simulink model "plant_control_2"  (R2023a)
settings: Solver=FixedStepAuto  StartTime=0.0  StopTime=10.0  FixedStep=0.01  RelTol=1e-3
values from neighbouring files (symbols this model uses):
  attitude_ref = [15, 10, 0]    [control_law_design.m]
  g = 9.81    [control_law_design.m]
  Kp_p = 0.4858    [control_law_design.m]
  Kp_pitch = 14    [control_law_design.m]
  Kp_q = 0.4858    [control_law_design.m]
  Kp_r = 0.881    [control_law_design.m]
  Kp_roll = 14    [control_law_design.m]
  Kp_yaw = 12    [control_law_design.m]
  m = 0.468    [control_law_design.m]
libraries: simulink_extras x2, shared6dof x1
settings Model: Creator=timme  LastModifiedBy=timme
settings OptimizationCC: BlockReduction=off  DefaultParameterBehavior=Inlined  BufferReuse=off

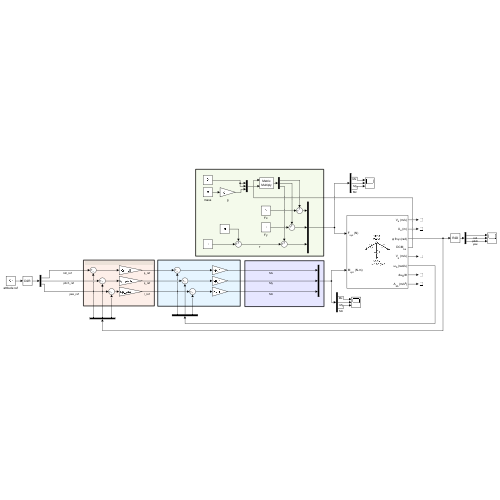
[thumbnail: Simulink's stored preview of the top-level diagram]
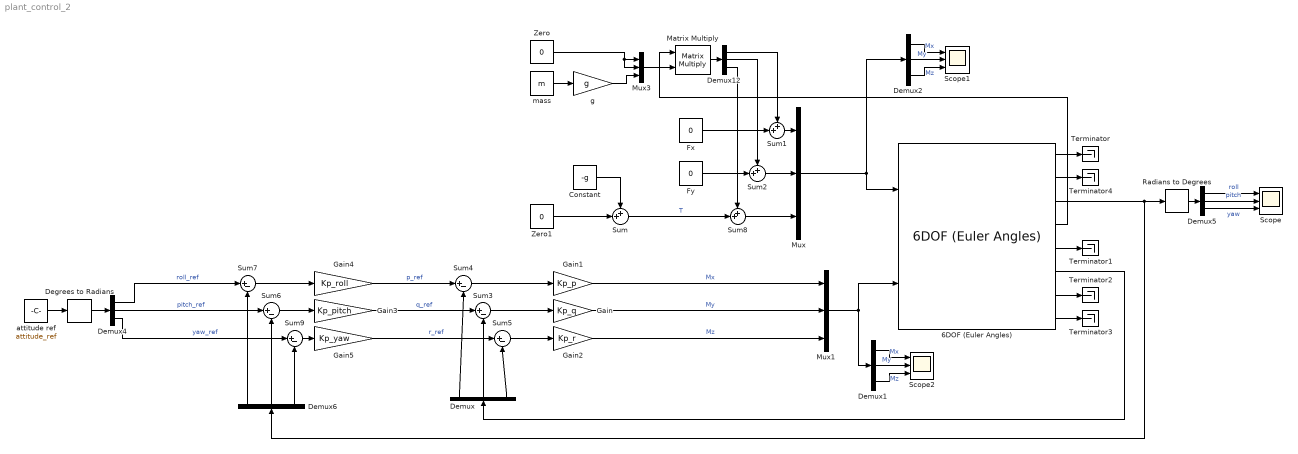
== system plant_control_2 ==
  6DOF (Euler Angles) : shared6dof/6DOF (Euler Angles)  units=Metric (MKS)  mtype=Fixed  rep=Euler Angles  xme_0=[0 0 0]  Vm_0=[0 0 0]  eul_0=[0 0 0]  pm_0=[0 0 0]  mass_0=m  mass_e=0.5  mass_f=2.0  inertia=I  inertia_e=eye(3)  inertia_f=2*eye(3)  k_quat=1.0  vre_flag=on  abi_flag=off  aMode=0  xme_statename=''  Vm_statename=''  eul_statename=''  quat_statename=''  pm_statename=''  mass_statename=''
  Constant : Constant  Value=-g
  Degrees to Radians : simulink_extras/Transformations/Degrees to Radians
  Demux{,1..2,4..6,12} (7 alike) : Demux  Outputs=3
  Fx : Constant  Value=0
  Fy : Constant  Value=0
  Gain : Gain  Gain=Kp_q
  Gain1 : Gain  Gain=Kp_p
  Gain2 : Gain  Gain=Kp_r
  Gain3 : Gain  Gain=Kp_pitch
  Gain4 : Gain  Gain=Kp_roll
  Gain5 : Gain  Gain=Kp_yaw
  Matrix Multiply : Product  Inputs=**  Multiplication=Matrix(*)
  Mux : Mux  Inputs=3
  Mux1 : Mux  Inputs=3
  Mux3 : Mux  Inputs=3
  Radians to Degrees : simulink_extras/Transformations/Radians to Degrees
  Scope : Scope  NumInputPorts=3
  Scope1 : Scope  NumInputPorts=3
  Scope2 : Scope  NumInputPorts=3
  Sum{,1..2,8} (4 alike) : Sum  Inputs=++|
  Sum{3..7,9} (6 alike) : Sum  Inputs=|+-
  Terminator{,1..4} (5 alike) : Terminator
  Zero : Constant  Value=0  OutDataTypeStr=Inherit: Inherit via back propagation
  Zero1 : Constant  Value=0  OutDataTypeStr=Inherit: Inherit via back propagation
  attitude ref : Constant  Value=attitude_ref
  g : Gain  Gain=g
  mass : Constant  Value=m
  wires:
  Mux1/1 -> 6DOF (Euler Angles)/2, Demux1/1
  6DOF (Euler Angles)/5 -> Terminator1/1
  6DOF (Euler Angles)/7 -> Terminator2/1
  6DOF (Euler Angles)/8 -> Terminator3/1
  Demux1/2 -> Scope2/2  "My"
  Demux1/1 -> Scope2/1  "Mx"
  Demux1/3 -> Scope2/3  "Mz"
  Gain1/1 -> Mux1/1  "Mx"
  Gain/1 -> Mux1/2  "My"
  Zero1/1 -> Sum/2
  mass/1 -> g/1
  Zero/1 -> Mux3/1, Mux3/2
  Sum2/1 -> Mux/2
  6DOF (Euler Angles)/4 -> Matrix Multiply/1
  Fx/1 -> Sum1/2
  Demux12/1 -> Sum1/1
  g/1 -> Mux3/3
  Constant/1 -> Sum/1
  Sum8/1 -> Mux/3
  Matrix Multiply/1 -> Demux12/1
  Sum/1 -> Sum8/2  "T"
  Sum1/1 -> Mux/1
  Demux12/3 -> Sum8/1
  Fy/1 -> Sum2/2
  Mux3/1 -> Matrix Multiply/2
  Demux12/2 -> Sum2/1
  Mux/1 -> Demux2/1, 6DOF (Euler Angles)/1
  Demux2/1 -> Scope1/1  "Mx"
  Demux2/2 -> Scope1/2  "My"
  Demux2/3 -> Scope1/3  "Mz"
  Sum3/1 -> Gain/1
  Gain3/1 -> Sum3/1  "q_ref"
  Gain4/1 -> Sum4/1  "p_ref"
  Gain2/1 -> Mux1/3  "Mz"
  Sum4/1 -> Gain1/1
  Sum5/1 -> Gain2/1
  Gain5/1 -> Sum5/1  "r_ref"
  6DOF (Euler Angles)/3 -> Radians to Degrees/1, Demux6/1
  6DOF (Euler Angles)/1 -> Terminator/1
  6DOF (Euler Angles)/2 -> Terminator4/1
  Sum9/1 -> Gain5/1
  Sum6/1 -> Gain3/1
  Demux4/1 -> Sum7/1  "roll_ref"
  Sum7/1 -> Gain4/1
  Demux4/2 -> Sum6/1  "pitch_ref"
  Demux4/3 -> Sum9/1  "yaw_ref"
  attitude ref/1 -> Degrees to Radians/1
  Degrees to Radians/1 -> Demux4/1
  Demux5/2 -> Scope/2  "pitch"
  Demux5/3 -> Scope/3  "yaw"
  Demux5/1 -> Scope/1  "roll"
  Radians to Degrees/1 -> Demux5/1
  Demux/2 -> Sum3/2
  Demux/3 -> Sum5/2
  Demux/1 -> Sum4/2
  6DOF (Euler Angles)/6 -> Demux/1
  Demux6/3 -> Sum9/2
  Demux6/2 -> Sum6/2
  Demux6/1 -> Sum7/2
